simulink library "NSA_DEVS_SINKS"  (R2025a)
settings: Solver=VariableStepAuto  StartTime=0.0  StopTime=10.0  RelTol=1e-3
libraries: NSA_DEVS_MATH_OPERATIONS x1, NSA_DEVS_SOURCES x1, $bdroot x1, NSA_DEVS_LOGISTICS x1
settings Model: Creator=david  LastModifiedBy=peter
settings OptimizationCC: ReuseModelBlockBuffer=off
settings RTWCC: GPUComputeCapability=3.5

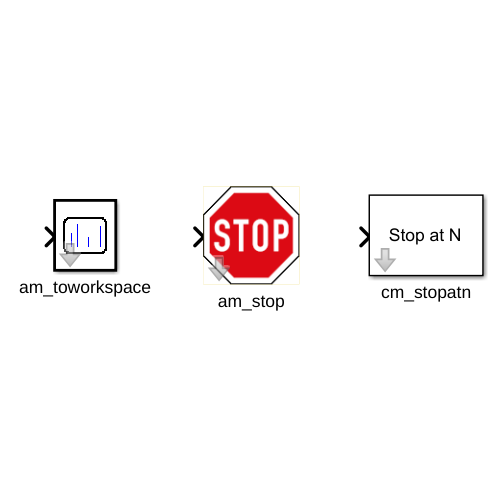
[thumbnail: Simulink's stored preview of the top-level diagram]
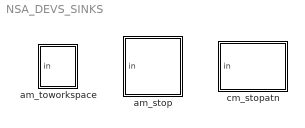
== system NSA_DEVS_SINKS ==
  am_stop : Subsystem  mask(Stop){tau=[0,1], debug=0}
      mask help: Terminates simulation when input is true.
      mask Help:
      | <p>Terminates simulation when input is true.</p>
      | 
      | <p>Ports
      | <ul>
      | <li>inputs:
      |   <ul>
      |     <li>in: incoming value</li>
      |   </ul>
      | </li>
      | <li>outputs:
      |   <ul>
      |     <li>-</li>
      |   </ul>
      | </li>
      | </ul>
      | </p>
      | 
      | <p>System Parameters
      |  <ul>
      | <li>name:  object name</li>
      | <li>debug: flag to enable debug information</li>
      | <li>tau:   infinitesimal delay</li>
      | </ul>
      | </p>
      | 
      | <p>States
      | <ul>
      | <li>s:   running</li>
      | </ul>
      | </p>
      mask DialogControl Container3 Prompt: Advanced
      mask Display: image('$imagefile'); % Use "Edit Image" on toolstrip to change.
  am_toworkspace : Subsystem  TreatAsAtomicUnit=on  mask(ToWorkspace){varname="varname", t0=0, format="vector", tau=[0,5], debug=0}
      mask help:
      | Stores time and value of incoming events in global variable
      |       simout.VARNAME in fields t and y
      mask Help:
      | <p>Stores time and value of incoming events in global variable
      |       simout.VARNAME in fields t and y</p>
      | <p>Ports
      | <ul>
      | <li>inputs:
      |   <ul>
      |     <li>in: incoming value</li>
      |   </ul>
      | </li>
      | <li>outputs: none</li>
      | </ul>
      | </p>
      | 
      | <p>System Parameters
      |  <ul>
      | <li>varname:  field name in global output variable</li>
      | <li>t0:  time of initial time stamp</li>
      | <li>format:  vector -> save x values in vector, single -> save the last value</li>
      | <li>debug: flag to enable debug information</li>
      | <li>tau:   infinitesimal delay</li>
      | </ul>
      | </p>
      | 
      |  <p>States
      | <ul>
      | <li>name:  object name</li>
      | <li>s:   running</li>
      | <li>t:  time of last event for time stamp</li>
      | </ul>
      | </p>
      mask TypeOptions format: "vector" | "single"
      mask DialogControl Container4 Prompt: General
      mask DialogControl Container5 Prompt: Advanced
      mask Display: image('icon_toworkspace.png');
  cm_stopatn : Subsystem  mask(StopAtN){N=10, tau=[0,1], debug=0}
      mask prompts: N "Number of entities to arrive before stop"
      mask help: Terminates simulation, when N entities have arrived.
      mask Help:
      | <p>Terminates simulation, when N entities have arrived.</p>
      | 
      | <p>Ports
      | <ul>
      | <li>inputs:
      |   <ul>
      |     <li>in: incoming entities</li>
      |   </ul>
      | </li>
      | </ul>
      | </p>
      | 
      | <p>System Parameters
      | <ul>
      | <li>N: Number of entities to arrive before stop</li>
      | <li>debug: flag to enable debug information</li>
      | <li>tau:   infinitesimal delay</li>
      | </ul>
      | </p>
      mask DialogControl Container4 Prompt: General
      mask DialogControl Container5 Prompt: Advanced
      mask Display: disp('Stop at N');

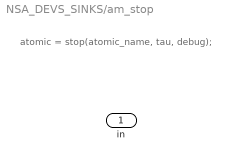
== system NSA_DEVS_SINKS/am_stop ==
  note: atomic = stop(atomic_name, tau, debug);
  in : Inport

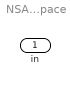
== system NSA_DEVS_SINKS/am_toworkspace ==
  in : Inport

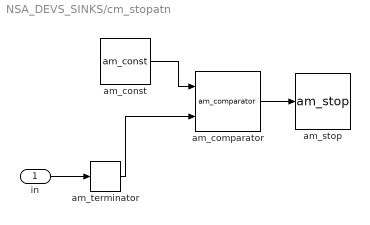
== system NSA_DEVS_SINKS/cm_stopatn ==
  in : Inport
  am_comparator : NSA_DEVS_MATH_OPERATIONS/am_comparator  compop="\"<=\""  tau=tau  debug=debug
      settings: SourceProductName=Math Operations
  am_const : NSA_DEVS_SOURCES/am_const  value=N  sendTime=[0,1]  debug=debug
      settings: SourceProductName=Sources
  am_stop : $bdroot/am_stop  tau=tau  debug=debug
  am_terminator : NSA_DEVS_LOGISTICS/am_terminator  tau=tau  debug=debug
      settings: SourceProductName=Logistics
  wires:
  am_comparator/1 -> am_stop/1
  am_terminator/1 -> am_comparator/2
  in/1 -> am_terminator/1
  am_const/1 -> am_comparator/1
